simulink model "s_cd_hmc_v3_dsim"  (R2016b)
(part 2 of 59)

      mask help:
      | An explicitly laid-out delay line to avoid mapping to SRL16s
      | for use in pipelining to help achieve timing closure.
      mask init:
      | pipeline_init(gcb,'latency',latency);
      settings: AttributesFormatString=Latency = %<latency>
      mask Display:
      | port_label('input', 1, 'd');
      | port_label('output', 1, 'q');
      | disp(['Z^-', num2str(latency)]);
  pipeline6 : Subsystem  AncestorBlock=casper_library_delays/pipeline  mask(pipeline){latency=2}
      mask help:
      | An explicitly laid-out delay line to avoid mapping to SRL16s
      | for use in pipelining to help achieve timing closure.
      mask init:
      | pipeline_init(gcb,'latency',latency);
      settings: AttributesFormatString=Latency = %<latency>
      mask Display:
      | port_label('input', 1, 'd');
      | port_label('output', 1, 'q');
      | disp(['Z^-', num2str(latency)]);
  pipeline60 : Subsystem  AncestorBlock=casper_library_delays/pipeline  mask(pipeline){latency=2}
      mask help:
      | An explicitly laid-out delay line to avoid mapping to SRL16s
      | for use in pipelining to help achieve timing closure.
      mask init:
      | pipeline_init(gcb,'latency',latency);
      settings: AttributesFormatString=Latency = %<latency>
      mask Display:
      | port_label('input', 1, 'd');
      | port_label('output', 1, 'q');
      | disp(['Z^-', num2str(latency)]);
  pipeline61 : Subsystem  AncestorBlock=casper_library_delays/pipeline  mask(pipeline){latency=2}
      mask help:
      | An explicitly laid-out delay line to avoid mapping to SRL16s
      | for use in pipelining to help achieve timing closure.
      mask init:
      | pipeline_init(gcb,'latency',latency);
      settings: AttributesFormatString=Latency = %<latency>
      mask Display:
      | port_label('input', 1, 'd');
      | port_label('output', 1, 'q');
      | disp(['Z^-', num2str(latency)]);
  pipeline62 : Subsystem  AncestorBlock=casper_library_delays/pipeline  mask(pipeline){latency=3}
      mask help:
      | An explicitly laid-out delay line to avoid mapping to SRL16s
      | for use in pipelining to help achieve timing closure.
      mask init:
      | pipeline_init(gcb,'latency',latency);
      settings: AttributesFormatString=Latency = %<latency>
      mask Display:
      | port_label('input', 1, 'd');
      | port_label('output', 1, 'q');
      | disp(['Z^-', num2str(latency)]);
  pipeline63 : Subsystem  AncestorBlock=casper_library_delays/pipeline  mask(pipeline){latency=2}
      mask help:
      | An explicitly laid-out delay line to avoid mapping to SRL16s
      | for use in pipelining to help achieve timing closure.
      mask init:
      | pipeline_init(gcb,'latency',latency);
      settings: AttributesFormatString=Latency = %<latency>
      mask Display:
      | port_label('input', 1, 'd');
      | port_label('output', 1, 'q');
      | disp(['Z^-', num2str(latency)]);
  pipeline64 : Subsystem  AncestorBlock=casper_library_delays/pipeline  mask(pipeline){latency=2}
      mask help:
      | An explicitly laid-out delay line to avoid mapping to SRL16s
      | for use in pipelining to help achieve timing closure.
      mask init:
      | pipeline_init(gcb,'latency',latency);
      settings: AttributesFormatString=Latency = %<latency>
      mask Display:
      | port_label('input', 1, 'd');
      | port_label('output', 1, 'q');
      | disp(['Z^-', num2str(latency)]);
  pipeline65 : Subsystem  AncestorBlock=casper_library_delays/pipeline  mask(pipeline){latency=3}
      mask help:
      | An explicitly laid-out delay line to avoid mapping to SRL16s
      | for use in pipelining to help achieve timing closure.
      mask init:
      | pipeline_init(gcb,'latency',latency);
      settings: AttributesFormatString=Latency = %<latency>
      mask Display:
      | port_label('input', 1, 'd');
      | port_label('output', 1, 'q');
      | disp(['Z^-', num2str(latency)]);
  pipeline66 : Subsystem  AncestorBlock=casper_library_delays/pipeline  mask(pipeline){latency=2}
      mask help:
      | An explicitly laid-out delay line to avoid mapping to SRL16s
      | for use in pipelining to help achieve timing closure.
      mask init:
      | pipeline_init(gcb,'latency',latency);
      settings: AttributesFormatString=Latency = %<latency>
      mask Display:
      | port_label('input', 1, 'd');
      | port_label('output', 1, 'q');
      | disp(['Z^-', num2str(latency)]);
  pipeline67 : Subsystem  AncestorBlock=casper_library_delays/pipeline  mask(pipeline){latency=2}
      mask help:
      | An explicitly laid-out delay line to avoid mapping to SRL16s
      | for use in pipelining to help achieve timing closure.
      mask init:
      | pipeline_init(gcb,'latency',latency);
      settings: AttributesFormatString=Latency = %<latency>
      mask Display:
      | port_label('input', 1, 'd');
      | port_label('output', 1, 'q');
      | disp(['Z^-', num2str(latency)]);
  pipeline68 : Subsystem  AncestorBlock=casper_library_delays/pipeline  mask(pipeline){latency=2}
      mask help:
      | An explicitly laid-out delay line to avoid mapping to SRL16s
      | for use in pipelining to help achieve timing closure.
      mask init:
      | pipeline_init(gcb,'latency',latency);
      settings: AttributesFormatString=Latency = %<latency>
      mask Display:
      | port_label('input', 1, 'd');
      | port_label('output', 1, 'q');
      | disp(['Z^-', num2str(latency)]);
  pipeline69 : Subsystem  AncestorBlock=casper_library_delays/pipeline  mask(pipeline){latency=2}
      mask help:
      | An explicitly laid-out delay line to avoid mapping to SRL16s
      | for use in pipelining to help achieve timing closure.
      mask init:
      | pipeline_init(gcb,'latency',latency);
      settings: AttributesFormatString=Latency = %<latency>
      mask Display:
      | port_label('input', 1, 'd');
      | port_label('output', 1, 'q');
      | disp(['Z^-', num2str(latency)]);
  pipeline7 : Subsystem  AncestorBlock=casper_library_delays/pipeline  mask(pipeline){latency=2}
      mask help:
      | An explicitly laid-out delay line to avoid mapping to SRL16s
      | for use in pipelining to help achieve timing closure.
      mask init:
      | pipeline_init(gcb,'latency',latency);
      settings: AttributesFormatString=Latency = %<latency>
      mask Display:
      | port_label('input', 1, 'd');
      | port_label('output', 1, 'q');
      | disp(['Z^-', num2str(latency)]);
  pipeline70 : Subsystem  AncestorBlock=casper_library_delays/pipeline  mask(pipeline){latency=2}
      mask help:
      | An explicitly laid-out delay line to avoid mapping to SRL16s
      | for use in pipelining to help achieve timing closure.
      mask init:
      | pipeline_init(gcb,'latency',latency);
      settings: AttributesFormatString=Latency = %<latency>
      mask Display:
      | port_label('input', 1, 'd');
      | port_label('output', 1, 'q');
      | disp(['Z^-', num2str(latency)]);
  pipeline71 : Subsystem  AncestorBlock=casper_library_delays/pipeline  mask(pipeline){latency=2}
      mask help:
      | An explicitly laid-out delay line to avoid mapping to SRL16s
      | for use in pipelining to help achieve timing closure.
      mask init:
      | pipeline_init(gcb,'latency',latency);
      settings: AttributesFormatString=Latency = %<latency>
      mask Display:
      | port_label('input', 1, 'd');
      | port_label('output', 1, 'q');
      | disp(['Z^-', num2str(latency)]);
  pipeline72 : Subsystem  AncestorBlock=casper_library_delays/pipeline  mask(pipeline){latency=1}
      mask help:
      | An explicitly laid-out delay line to avoid mapping to SRL16s
      | for use in pipelining to help achieve timing closure.
      mask init:
      | pipeline_init(gcb,'latency',latency);
      settings: AttributesFormatString=Latency = %<latency>
      mask Display:
      | port_label('input', 1, 'd');
      | port_label('output', 1, 'q');
      | disp(['Z^-', num2str(latency)]);
  pipeline74 : Subsystem  AncestorBlock=casper_library_delays/pipeline  mask(pipeline){latency=2}
      mask help:
      | An explicitly laid-out delay line to avoid mapping to SRL16s
      | for use in pipelining to help achieve timing closure.
      mask init:
      | pipeline_init(gcb,'latency',latency);
      settings: AttributesFormatString=Latency = %<latency>
      mask Display:
      | port_label('input', 1, 'd');
      | port_label('output', 1, 'q');
      | disp(['Z^-', num2str(latency)]);
  pipeline75 : Subsystem  AncestorBlock=casper_library_delays/pipeline  mask(pipeline){latency=2}
      mask help:
      | An explicitly laid-out delay line to avoid mapping to SRL16s
      | for use in pipelining to help achieve timing closure.
      mask init:
      | pipeline_init(gcb,'latency',latency);
      settings: AttributesFormatString=Latency = %<latency>
      mask Display:
      | port_label('input', 1, 'd');
      | port_label('output', 1, 'q');
      | disp(['Z^-', num2str(latency)]);
  pipeline76 : Subsystem  AncestorBlock=casper_library_delays/pipeline  mask(pipeline){latency=2}
      mask help:
      | An explicitly laid-out delay line to avoid mapping to SRL16s
      | for use in pipelining to help achieve timing closure.
      mask init:
      | pipeline_init(gcb,'latency',latency);
      settings: AttributesFormatString=Latency = %<latency>
      mask Display:
      | port_label('input', 1, 'd');
      | port_label('output', 1, 'q');
      | disp(['Z^-', num2str(latency)]);
  pipeline79 : Subsystem  AncestorBlock=casper_library_delays/pipeline  mask(pipeline){latency=2}
      mask help:
      | An explicitly laid-out delay line to avoid mapping to SRL16s
      | for use in pipelining to help achieve timing closure.
      mask init:
      | pipeline_init(gcb,'latency',latency);
      settings: AttributesFormatString=Latency = %<latency>
      mask Display:
      | port_label('input', 1, 'd');
      | port_label('output', 1, 'q');
      | disp(['Z^-', num2str(latency)]);
  pipeline8 : Subsystem  AncestorBlock=casper_library_delays/pipeline  mask(pipeline){latency=2}
      mask help:
      | An explicitly laid-out delay line to avoid mapping to SRL16s
      | for use in pipelining to help achieve timing closure.
      mask init:
      | pipeline_init(gcb,'latency',latency);
      settings: AttributesFormatString=Latency = %<latency>
      mask Display:
      | port_label('input', 1, 'd');
      | port_label('output', 1, 'q');
      | disp(['Z^-', num2str(latency)]);
  pipeline80 : Subsystem  AncestorBlock=casper_library_delays/pipeline  mask(pipeline){latency=2}
      mask help:
      | An explicitly laid-out delay line to avoid mapping to SRL16s
      | for use in pipelining to help achieve timing closure.
      mask init:
      | pipeline_init(gcb,'latency',latency);
      settings: AttributesFormatString=Latency = %<latency>
      mask Display:
      | port_label('input', 1, 'd');
      | port_label('output', 1, 'q');
      | disp(['Z^-', num2str(latency)]);
  pipeline81 : Subsystem  AncestorBlock=casper_library_delays/pipeline  mask(pipeline){latency=2}
      mask help:
      | An explicitly laid-out delay line to avoid mapping to SRL16s
      | for use in pipelining to help achieve timing closure.
      mask init:
      | pipeline_init(gcb,'latency',latency);
      settings: AttributesFormatString=Latency = %<latency>
      mask Display:
      | port_label('input', 1, 'd');
      | port_label('output', 1, 'q');
      | disp(['Z^-', num2str(latency)]);
  pipeline82 : Subsystem  AncestorBlock=casper_library_delays/pipeline  mask(pipeline){latency=2}
      mask help:
      | An explicitly laid-out delay line to avoid mapping to SRL16s
      | for use in pipelining to help achieve timing closure.
      mask init:
      | pipeline_init(gcb,'latency',latency);
      settings: AttributesFormatString=Latency = %<latency>
      mask Display:
      | port_label('input', 1, 'd');
      | port_label('output', 1, 'q');
      | disp(['Z^-', num2str(latency)]);
  pipeline83 : Subsystem  AncestorBlock=casper_library_delays/pipeline  mask(pipeline){latency=2}
      mask help:
      | An explicitly laid-out delay line to avoid mapping to SRL16s
      | for use in pipelining to help achieve timing closure.
      mask init:
      | pipeline_init(gcb,'latency',latency);
      settings: AttributesFormatString=Latency = %<latency>
      mask Display:
      | port_label('input', 1, 'd');
      | port_label('output', 1, 'q');
      | disp(['Z^-', num2str(latency)]);
  pipeline85 : Subsystem  AncestorBlock=casper_library_delays/pipeline  mask(pipeline){latency=2}
      mask help:
      | An explicitly laid-out delay line to avoid mapping to SRL16s
      | for use in pipelining to help achieve timing closure.
      mask init:
      | pipeline_init(gcb,'latency',latency);
      settings: AttributesFormatString=Latency = %<latency>
      mask Display:
      | port_label('input', 1, 'd');
      | port_label('output', 1, 'q');
      | disp(['Z^-', num2str(latency)]);
  pipeline86 : Subsystem  AncestorBlock=casper_library_delays/pipeline  mask(pipeline){latency=2}
      mask help:
      | An explicitly laid-out delay line to avoid mapping to SRL16s
      | for use in pipelining to help achieve timing closure.
      mask init:
      | pipeline_init(gcb,'latency',latency);
      settings: AttributesFormatString=Latency = %<latency>
      mask Display:
      | port_label('input', 1, 'd');
      | port_label('output', 1, 'q');
      | disp(['Z^-', num2str(latency)]);
  pipeline87 : Subsystem  AncestorBlock=casper_library_delays/pipeline  mask(pipeline){latency=2}
      mask help:
      | An explicitly laid-out delay line to avoid mapping to SRL16s
      | for use in pipelining to help achieve timing closure.
      mask init:
      | pipeline_init(gcb,'latency',latency);
      settings: AttributesFormatString=Latency = %<latency>
      mask Display:
      | port_label('input', 1, 'd');
      | port_label('output', 1, 'q');
      | disp(['Z^-', num2str(latency)]);
  pipeline9 : Subsystem  AncestorBlock=casper_library_delays/pipeline  mask(pipeline){latency=2}
      mask help:
      | An explicitly laid-out delay line to avoid mapping to SRL16s
      | for use in pipelining to help achieve timing closure.
      mask init:
      | pipeline_init(gcb,'latency',latency);
      settings: AttributesFormatString=Latency = %<latency>
      mask Display:
      | port_label('input', 1, 'd');
      | port_label('output', 1, 'q');
      | disp(['Z^-', num2str(latency)]);
  pipeline90 : Subsystem  AncestorBlock=casper_library_delays/pipeline  mask(pipeline){latency=2}
      mask help:
      | An explicitly laid-out delay line to avoid mapping to SRL16s
      | for use in pipelining to help achieve timing closure.
      mask init:
      | pipeline_init(gcb,'latency',latency);
      settings: AttributesFormatString=Latency = %<latency>
      mask Display:
      | port_label('input', 1, 'd');
      | port_label('output', 1, 'q');
      | disp(['Z^-', num2str(latency)]);
  pipeline91 : Subsystem  AncestorBlock=casper_library_delays/pipeline  mask(pipeline){latency=2}
      mask help:
      | An explicitly laid-out delay line to avoid mapping to SRL16s
      | for use in pipelining to help achieve timing closure.
      mask init:
      | pipeline_init(gcb,'latency',latency);
      settings: AttributesFormatString=Latency = %<latency>
      mask Display:
      | port_label('input', 1, 'd');
      | port_label('output', 1, 'q');
      | disp(['Z^-', num2str(latency)]);
  pipeline92 : Subsystem  AncestorBlock=casper_library_delays/pipeline  mask(pipeline){latency=2}
      mask help:
      | An explicitly laid-out delay line to avoid mapping to SRL16s
      | for use in pipelining to help achieve timing closure.
      mask init:
      | pipeline_init(gcb,'latency',latency);
      settings: AttributesFormatString=Latency = %<latency>
      mask Display:
      | port_label('input', 1, 'd');
      | port_label('output', 1, 'q');
      | disp(['Z^-', num2str(latency)]);
  pipeline93 : Subsystem  AncestorBlock=casper_library_delays/pipeline  mask(pipeline){latency=2}
      mask help:
      | An explicitly laid-out delay line to avoid mapping to SRL16s
      | for use in pipelining to help achieve timing closure.
      mask init:
      | pipeline_init(gcb,'latency',latency);
      settings: AttributesFormatString=Latency = %<latency>
      mask Display:
      | port_label('input', 1, 'd');
      | port_label('output', 1, 'q');
      | disp(['Z^-', num2str(latency)]);
  pipeline94 : Subsystem  AncestorBlock=casper_library_delays/pipeline  mask(pipeline){latency=2}
      mask help:
      | An explicitly laid-out delay line to avoid mapping to SRL16s
      | for use in pipelining to help achieve timing closure.
      mask init:
      | pipeline_init(gcb,'latency',latency);
      settings: AttributesFormatString=Latency = %<latency>
      mask Display:
      | port_label('input', 1, 'd');
      | port_label('output', 1, 'q');
      | disp(['Z^-', num2str(latency)]);
  pipeline95 : Subsystem  AncestorBlock=casper_library_delays/pipeline  mask(pipeline){latency=2}
      mask help:
      | An explicitly laid-out delay line to avoid mapping to SRL16s
      | for use in pipelining to help achieve timing closure.
      mask init:
      | pipeline_init(gcb,'latency',latency);
      settings: AttributesFormatString=Latency = %<latency>
      mask Display:
      | port_label('input', 1, 'd');
      | port_label('output', 1, 'q');
      | disp(['Z^-', num2str(latency)]);
  pipeline96 : Subsystem  AncestorBlock=casper_library_delays/pipeline  mask(pipeline){latency=2}
      mask help:
      | An explicitly laid-out delay line to avoid mapping to SRL16s
      | for use in pipelining to help achieve timing closure.
      mask init:
      | pipeline_init(gcb,'latency',latency);
      settings: AttributesFormatString=Latency = %<latency>
      mask Display:
      | port_label('input', 1, 'd');
      | port_label('output', 1, 'q');
      | disp(['Z^-', num2str(latency)]);
  pipeline97 : Subsystem  AncestorBlock=casper_library_delays/pipeline  mask(pipeline){latency=2}
      mask help:
      | An explicitly laid-out delay line to avoid mapping to SRL16s
      | for use in pipelining to help achieve timing closure.
      mask init:
      | pipeline_init(gcb,'latency',latency);
      settings: AttributesFormatString=Latency = %<latency>
      mask Display:
      | port_label('input', 1, 'd');
      | port_label('output', 1, 'q');
      | disp(['Z^-', num2str(latency)]);
  pipeline98 : Subsystem  AncestorBlock=casper_library_delays/pipeline  mask(pipeline){latency=2}
      mask help:
      | An explicitly laid-out delay line to avoid mapping to SRL16s
      | for use in pipelining to help achieve timing closure.
      mask init:
      | pipeline_init(gcb,'latency',latency);
      settings: AttributesFormatString=Latency = %<latency>
      mask Display:
      | port_label('input', 1, 'd');
      | port_label('output', 1, 'q');
      | disp(['Z^-', num2str(latency)]);
  pipeline99 : Subsystem  AncestorBlock=casper_library_delays/pipeline  mask(pipeline){latency=2}
      mask help:
      | An explicitly laid-out delay line to avoid mapping to SRL16s
      | for use in pipelining to help achieve timing closure.
      mask init:
      | pipeline_init(gcb,'latency',latency);
      settings: AttributesFormatString=Latency = %<latency>
      mask Display:
      | port_label('input', 1, 'd');
      | port_label('output', 1, 'q');
      | disp(['Z^-', num2str(latency)]);
  reorder_status : Subsystem  Tag=xps:sw_reg  AncestorBlock=xps_library/software_register  mask(swreg){io_dir=To Processor, io_delay=0, sample_period=1, names=[timestep_err_cnt receive_err_cnt discard_cnt relock_err_cnt overflow_err_cnt], bitwidths=5, bin_pts=0, arith_types=0, sim_port=off, show_format=on}
      mask prompts: io_dir "I/O direction"; io_delay "I/O delay"; sample_period "Sample period"; names "Bitfield names [msb...lsb]"; bitwidths "Bitfield widths"; bin_pts "Bitfield binary pts"; arith_types "Bitfield types, ufix=0, fix=1, bool=2"; sim_port "Provide sim input/output?"; show_format "Print format string?"
      mask help: A 32-bit software-accessible register. Can be divided into bitfields of varying widths and types using the fields in the block mask.
      mask init:
      | swreg_init(gcb)
      settings: AttributesFormatString=5 outputs:uf5.0,uf5.0,uf5.0,uf5.0,uf5.0 = 25 bits
      mask TypeOptions io_dir: To Processor | From Processor
      mask Callback io_dir:
      | mask_enables = get_param(gcb, 'MaskEnables');
      | mask_names = get_param(gcb, 'MaskNames');
      | if strcmp(get_param(gcb, 'io_dir'), 'To Processor'),
      |     mask_enables{ismember(mask_names, 'sample_period')} = 'off';
      | else
      |     mask_enables{ismember(mask_names, 'sample_period')} = 'on';
      | end
      | set_param(gcb, 'MaskEnables', mask_enables);
  rx_dest_ip : Subsystem  Tag=xps:sw_reg  AncestorBlock=xps_library/software register  mask(swreg){io_dir=To Processor, io_delay=0, sample_period=1, names=reg, bitwidths=32, bin_pts=0, arith_types=0, sim_port=off, show_format=on}
      mask prompts: io_dir "I/O direction"; io_delay "I/O delay"; sample_period "Sample period"; names "Bitfield names [msb...lsb]"; bitwidths "Bitfield widths"; bin_pts "Bitfield binary pts"; arith_types "Bitfield types, ufix=0, fix=1, bool=2"; sim_port "Provide sim input/output?"; show_format "Print format string?"
      mask help: A 32-bit software-accessible register. Can be divided into bitfields of varying widths and types using the fields in the block mask.
      mask init:
      | swreg_init(gcb)
      settings: AttributesFormatString=1output:uf32.0 = 32 bits
      mask TypeOptions io_dir: To Processor | From Processor
      mask Callback io_dir:
      | mask_enables = get_param(gcb, 'MaskEnables');
      | mask_names = get_param(gcb, 'MaskNames');
      | if strcmp(get_param(gcb, 'io_dir'), 'To Processor'),
      |     mask_enables{ismember(mask_names, 'sample_period')} = 'off';
      | else
      |     mask_enables{ismember(mask_names, 'sample_period')} = 'on';
      | end
      | set_param(gcb, 'MaskEnables', mask_enables);
  rx_dest_port : Subsystem  Tag=xps:sw_reg  AncestorBlock=xps_library/software register  mask(swreg){io_dir=To Processor, io_delay=0, sample_period=1, names=reg, bitwidths=16, bin_pts=0, arith_types=0, sim_port=off, show_format=on}
      mask prompts: io_dir "I/O direction"; io_delay "I/O delay"; sample_period "Sample period"; names "Bitfield names [msb...lsb]"; bitwidths "Bitfield widths"; bin_pts "Bitfield binary pts"; arith_types "Bitfield types, ufix=0, fix=1, bool=2"; sim_port "Provide sim input/output?"; show_format "Print format string?"
      mask help: A 32-bit software-accessible register. Can be divided into bitfields of varying widths and types using the fields in the block mask.
      mask init:
      | swreg_init(gcb)
      settings: AttributesFormatString=1output:uf16.0 = 16 bits
      mask TypeOptions io_dir: To Processor | From Processor
      mask Callback io_dir:
      | mask_enables = get_param(gcb, 'MaskEnables');
      | mask_names = get_param(gcb, 'MaskNames');
      | if strcmp(get_param(gcb, 'io_dir'), 'To Processor'),
      |     mask_enables{ismember(mask_names, 'sample_period')} = 'off';
      | else
      |     mask_enables{ismember(mask_names, 'sample_period')} = 'on';
      | end
      | set_param(gcb, 'MaskEnables', mask_enables);
  rx_src_ip : Subsystem  Tag=xps:sw_reg  AncestorBlock=xps_library/software register  mask(swreg){io_dir=To Processor, io_delay=0, sample_period=1, names=reg, bitwidths=32, bin_pts=0, arith_types=0, sim_port=off, show_format=on}
      mask prompts: io_dir "I/O direction"; io_delay "I/O delay"; sample_period "Sample period"; names "Bitfield names [msb...lsb]"; bitwidths "Bitfield widths"; bin_pts "Bitfield binary pts"; arith_types "Bitfield types, ufix=0, fix=1, bool=2"; sim_port "Provide sim input/output?"; show_format "Print format string?"
      mask help: A 32-bit software-accessible register. Can be divided into bitfields of varying widths and types using the fields in the block mask.
      mask init:
      | swreg_init(gcb)
      settings: AttributesFormatString=1output:uf32.0 = 32 bits
      mask TypeOptions io_dir: To Processor | From Processor
      mask Callback io_dir:
      | mask_enables = get_param(gcb, 'MaskEnables');
      | mask_names = get_param(gcb, 'MaskNames');
      | if strcmp(get_param(gcb, 'io_dir'), 'To Processor'),
      |     mask_enables{ismember(mask_names, 'sample_period')} = 'off';
      | else
      |     mask_enables{ismember(mask_names, 'sample_period')} = 'on';
      | end
      | set_param(gcb, 'MaskEnables', mask_enables);
  rx_src_port : Subsystem  Tag=xps:sw_reg  AncestorBlock=xps_library/software register  mask(swreg){io_dir=To Processor, io_delay=0, sample_period=1, names=reg, bitwidths=16, bin_pts=0, arith_types=0, sim_port=off, show_format=on}
      mask prompts: io_dir "I/O direction"; io_delay "I/O delay"; sample_period "Sample period"; names "Bitfield names [msb...lsb]"; bitwidths "Bitfield widths"; bin_pts "Bitfield binary pts"; arith_types "Bitfield types, ufix=0, fix=1, bool=2"; sim_port "Provide sim input/output?"; show_format "Print format string?"
      mask help: A 32-bit software-accessible register. Can be divided into bitfields of varying widths and types using the fields in the block mask.
      mask init:
      | swreg_init(gcb)
      settings: AttributesFormatString=1output:uf16.0 = 16 bits
      mask TypeOptions io_dir: To Processor | From Processor
      mask Callback io_dir:
      | mask_enables = get_param(gcb, 'MaskEnables');
      | mask_names = get_param(gcb, 'MaskNames');
      | if strcmp(get_param(gcb, 'io_dir'), 'To Processor'),
      |     mask_enables{ismember(mask_names, 'sample_period')} = 'off';
      | else
      |     mask_enables{ismember(mask_names, 'sample_period')} = 'on';
      | end
      | set_param(gcb, 'MaskEnables', mask_enables);
  snap_adc0 : Subsystem  Tag=casper:bitsnap  AncestorBlock=casper_library_scopes/bitfield snapshot  mask(bitsnap){io_names=[d0 d1 d2 d3 d4 d5 d6 d7 dv sync], io_widths=[10 10 10 10 10 10 10 10 1 1], io_bps=[9 9 9 9 9 9 9 9 0 0], io_types=[1 1 1 1 1 1 1 1 2 2], snap_storage=bram, snap_dram_dimm=2, snap_dram_clock=250, snap_nsamples=11, snap_data_width=128, snap_offset=on, snap_circap=off, snap_value=off, snap_use_dsp48=off, snap_delay=0, extra_names=[c d], extra_widths=[30 2], extra_bps=[0 0], extra_types=[0 0]}
      mask prompts: io_names "Names [msb...lsb]"; io_widths "Widths [msb...lsb]"; io_bps "Binary pts [msb...lsb]"; io_types "Data types [msb...lsb], ufix=0, fix=1, bool=2"; snap_storage "Storage medium"; snap_dram_dimm "DRAM dimm"; snap_dram_clock "DRAM clock rate"; snap_nsamples "Number of Samples (2^?)"; snap_data_width "Data width"; snap_offset "Start delay support"; snap_circap "Circular capture support"; snap_value "Extra value capture support"; snap_use_dsp48 "Use DSP48s to implement counters"; snap_delay "Pre-snapshot delay"; extra_names "Names [msb...lsb]"; extra_widths "Widths [msb...lsb]"; extra_bps "Binary pts [msb...lsb]"; extra_types "Data types [msb...lsb], ufix=0, fix=1, bool=2"
      mask help:
      | A wrapped snapshot block. Allows specification of inputs to a snapblock word so the toolflow can automatically set up the scope.
      | See documentation for snapshot for explanation of parameters.
      mask init:
      | bitsnap_init(gcb);
      mask TypeOptions snap_storage: bram | dram
      mask Callback snap_storage: bitsnap_callback();
      mask TypeOptions snap_dram_dimm: 1 | 2 | 3 | 4
      mask TypeOptions snap_dram_clock: 200 | 250 | 266 | 300 | 333
      mask TypeOptions snap_data_width: 8 | 16 | 32 | 64 | 128
      mask Callback snap_value: bitsnap_callback();
  snap_adc1 : Subsystem  Tag=casper:bitsnap  AncestorBlock=casper_library_scopes/bitfield snapshot  mask(bitsnap){io_names=[d0 d1 d2 d3 d4 d5 d6 d7 dv sync], io_widths=[10 10 10 10 10 10 10 10 1 1], io_bps=[9 9 9 9 9 9 9 9 0 0], io_types=[1 1 1 1 1 1 1 1 2 2], snap_storage=bram, snap_dram_dimm=2, snap_dram_clock=250, snap_nsamples=11, snap_data_width=128, snap_offset=on, snap_circap=off, snap_value=off, snap_use_dsp48=off, snap_delay=0, extra_names=[c d], extra_widths=[30 2], extra_bps=[0 0], extra_types=[0 0]}
      mask prompts: io_names "Names [msb...lsb]"; io_widths "Widths [msb...lsb]"; io_bps "Binary pts [msb...lsb]"; io_types "Data types [msb...lsb], ufix=0, fix=1, bool=2"; snap_storage "Storage medium"; snap_dram_dimm "DRAM dimm"; snap_dram_clock "DRAM clock rate"; snap_nsamples "Number of Samples (2^?)"; snap_data_width "Data width"; snap_offset "Start delay support"; snap_circap "Circular capture support"; snap_value "Extra value capture support"; snap_use_dsp48 "Use DSP48s to implement counters"; snap_delay "Pre-snapshot delay"; extra_names "Names [msb...lsb]"; extra_widths "Widths [msb...lsb]"; extra_bps "Binary pts [msb...lsb]"; extra_types "Data types [msb...lsb], ufix=0, fix=1, bool=2"
      mask help:
      | A wrapped snapshot block. Allows specification of inputs to a snapblock word so the toolflow can automatically set up the scope.
      | See documentation for snapshot for explanation of parameters.
      mask init:
      | bitsnap_init(gcb);
      mask TypeOptions snap_storage: bram | dram
      mask Callback snap_storage: bitsnap_callback();
      mask TypeOptions snap_dram_dimm: 1 | 2 | 3 | 4
      mask TypeOptions snap_dram_clock: 200 | 250 | 266 | 300 | 333
      mask TypeOptions snap_data_width: 8 | 16 | 32 | 64 | 128
      mask Callback snap_value: bitsnap_callback();
  spead_status : Subsystem  Tag=xps:sw_reg  AncestorBlock=xps_library/software_register  mask(swreg){io_dir=To Processor, io_delay=0, sample_period=1, names=[magic_err_cnt header_err_cnt pad_err_cnt pkt_len_err_cnt pkt_cnt], bitwidths=6, bin_pts=0, arith_types=0, sim_port=off, show_format=on}
      mask prompts: io_dir "I/O direction"; io_delay "I/O delay"; sample_period "Sample period"; names "Bitfield names [msb...lsb]"; bitwidths "Bitfield widths"; bin_pts "Bitfield binary pts"; arith_types "Bitfield types, ufix=0, fix=1, bool=2"; sim_port "Provide sim input/output?"; show_format "Print format string?"
      mask help: A 32-bit software-accessible register. Can be divided into bitfields of varying widths and types using the fields in the block mask.
      mask init:
      | swreg_init(gcb)
      settings: AttributesFormatString=5 outputs:uf6.0,uf6.0,uf6.0,uf6.0,uf6.0 = 30 bits
      mask TypeOptions io_dir: To Processor | From Processor
      mask Callback io_dir:
      | mask_enables = get_param(gcb, 'MaskEnables');
      | mask_names = get_param(gcb, 'MaskNames');
      | if strcmp(get_param(gcb, 'io_dir'), 'To Processor'),
      |     mask_enables{ismember(mask_names, 'sample_period')} = 'off';
      | else
      |     mask_enables{ismember(mask_names, 'sample_period')} = 'on';
      | end
      | set_param(gcb, 'MaskEnables', mask_enables);
  sync_gen : Subsystem  mask{zerolsbs=((15 + 1) + 8)}
      mask prompts: zerolsbs "No. LSBs to be zero:"
  sys_rst_cnt : Subsystem  Tag=xps:sw_reg  AncestorBlock=xps_library/software register  mask(swreg){io_dir=To Processor, io_delay=0, sample_period=1, names=cnt, bitwidths=32, bin_pts=0, arith_types=0, sim_port=off, show_format=on}
      mask prompts: io_dir "I/O direction"; io_delay "I/O delay"; sample_period "Sample period"; names "Bitfield names [msb...lsb]"; bitwidths "Bitfield widths"; bin_pts "Bitfield binary pts"; arith_types "Bitfield types, ufix=0, fix=1, bool=2"; sim_port "Provide sim input/output?"; show_format "Print format string?"
      mask help: A 32-bit software-accessible register. Can be divided into bitfields of varying widths and types using the fields in the block mask.
      mask init:
      | swreg_init(gcb)
      settings: AttributesFormatString=1output:uf32.0 = 32 bits
      mask TypeOptions io_dir: To Processor | From Processor
      mask Callback io_dir:
      | mask_enables = get_param(gcb, 'MaskEnables');
      | mask_names = get_param(gcb, 'MaskNames');
      | if strcmp(get_param(gcb, 'io_dir'), 'To Processor'),
      |     mask_enables{ismember(mask_names, 'sample_period')} = 'off';
      | else
      |     mask_enables{ismember(mask_names, 'sample_period')} = 'on';
      | end
      | set_param(gcb, 'MaskEnables', mask_enables);
  time_gen1 : Subsystem  mask{n_bits_period=fft_stages-1-2-1+8, n_bits_increment=0, n_bits_counter=48-(fft_stages+8)}
      mask prompts: n_bits_period "Period (2^?)"; n_bits_increment "Increment (2^?)"; n_bits_counter "Counter size (2^?)"
  time_gen_cd : Subsystem  mask{n_bits_period=fft_stages-1-2, n_bits_increment=0, n_bits_counter=48-fft_stages}
      mask prompts: n_bits_period "Period (2^?)"; n_bits_increment "Increment (2^?)"; n_bits_counter "Counter size (2^?)"
  time_rst_cnt : Subsystem  Tag=xps:sw_reg  AncestorBlock=xps_library/software register  mask(swreg){io_dir=To Processor, io_delay=0, sample_period=1, names=cnt, bitwidths=32, bin_pts=0, arith_types=0, sim_port=off, show_format=on}
      mask prompts: io_dir "I/O direction"; io_delay "I/O delay"; sample_period "Sample period"; names "Bitfield names [msb...lsb]"; bitwidths "Bitfield widths"; bin_pts "Bitfield binary pts"; arith_types "Bitfield types, ufix=0, fix=1, bool=2"; sim_port "Provide sim input/output?"; show_format "Print format string?"
      mask help: A 32-bit software-accessible register. Can be divided into bitfields of varying widths and types using the fields in the block mask.
      mask init:
      | swreg_init(gcb)
      settings: AttributesFormatString=1output:uf32.0 = 32 bits
      mask TypeOptions io_dir: To Processor | From Processor
      mask Callback io_dir:
      | mask_enables = get_param(gcb, 'MaskEnables');
      | mask_names = get_param(gcb, 'MaskNames');
      | if strcmp(get_param(gcb, 'io_dir'), 'To Processor'),
      |     mask_enables{ismember(mask_names, 'sample_period')} = 'off';
      | else
      |     mask_enables{ismember(mask_names, 'sample_period')} = 'on';
      | end
      | set_param(gcb, 'MaskEnables', mask_enables);
  tl_cd0 : Subsystem  mask(timed_latch){n_bits_time=48-fft_stages, n_bits_quantization=fft_stages, n_bits_counters=4}
      mask prompts: n_bits_time "Number bits in time to compare"; n_bits_quantization "Time offset from lsb"; n_bits_counters "Bits in status counters"
      mask help:
      | Latches load_value when armed and current_time matches requested time.
      | current_time should be in ADC samples.
      mask init:
      | set_param([gcb,'/status'], 'bitwidths', mat2str([1, repmat(n_bits_counters, 1, 2)]));
      mask Help:
      | When armed, will latch new value when current time matches the time
      | specified. The input time should be in samples and mask settings allow
      | a portion of this to be compared to cater for quantization. Arm and latch
      | counts allow the current state, pending and missed latch events to be
      | determined.
  tl_cd0_control : Subsystem  Tag=xps:sw_reg  AncestorBlock=xps_library/software_register  mask(swreg){io_dir=From Processor, io_delay=0, sample_period=1, names=[arm load_immediate load_time_msw], bitwidths=[1 1 16], bin_pts=[0 0 0], arith_types=[2 2 0], sim_port=on, show_format=on}
      mask prompts: io_dir "I/O direction"; io_delay "I/O delay"; sample_period "Sample period"; names "Bitfield names [msb...lsb]"; bitwidths "Bitfield widths"; bin_pts "Bitfield binary pts"; arith_types "Bitfield types, ufix=0, fix=1, bool=2"; sim_port "Provide sim input/output?"; show_format "Print format string?"
      mask help: A 32-bit software-accessible register. Can be divided into bitfields of varying widths and types using the fields in the block mask.
      mask init:
      | swreg_init(gcb)
      settings: AttributesFormatString=3 inputs:b,b,uf16.0 = 18 bits
      mask TypeOptions io_dir: To Processor | From Processor
      mask Callback io_dir:
      | mask_enables = get_param(gcb, 'MaskEnables');
      | mask_names = get_param(gcb, 'MaskNames');
      | if strcmp(get_param(gcb, 'io_dir'), 'To Processor'),
      |     mask_enables{ismember(mask_names, 'sample_period')} = 'off';
      | else
      |     mask_enables{ismember(mask_names, 'sample_period')} = 'on';
      | end
      | set_param(gcb, 'MaskEnables', mask_enables);
  tl_cd0_control_lsw : Subsystem  Tag=xps:sw_reg  AncestorBlock=xps_library/software_register  mask(swreg){io_dir=From Processor, io_delay=0, sample_period=1, names=load_time_lsw, bitwidths=32, bin_pts=0, arith_types=0, sim_port=on, show_format=on}
      mask prompts: io_dir "I/O direction"; io_delay "I/O delay"; sample_period "Sample period"; names "Bitfield names [msb...lsb]"; bitwidths "Bitfield widths"; bin_pts "Bitfield binary pts"; arith_types "Bitfield types, ufix=0, fix=1, bool=2"; sim_port "Provide sim input/output?"; show_format "Print format string?"
      mask help: A 32-bit software-accessible register. Can be divided into bitfields of varying widths and types using the fields in the block mask.
      mask init:
      | swreg_init(gcb)
      settings: AttributesFormatString=1input:uf32.0 = 32 bits
      mask TypeOptions io_dir: To Processor | From Processor
      mask Callback io_dir:
      | mask_enables = get_param(gcb, 'MaskEnables');
      | mask_names = get_param(gcb, 'MaskNames');
      | if strcmp(get_param(gcb, 'io_dir'), 'To Processor'),
      |     mask_enables{ismember(mask_names, 'sample_period')} = 'off';
      | else
      |     mask_enables{ismember(mask_names, 'sample_period')} = 'on';
      | end
      | set_param(gcb, 'MaskEnables', mask_enables);
  tl_cd1 : Subsystem  mask(timed_latch){n_bits_time=48-fft_stages, n_bits_quantization=fft_stages, n_bits_counters=4}
      mask prompts: n_bits_time "Number bits in time to compare"; n_bits_quantization "Time offset from lsb"; n_bits_counters "Bits in status counters"
      mask help:
      | Latches load_value when armed and current_time matches requested time.
      | current_time should be in ADC samples.
      mask init:
      | set_param([gcb,'/status'], 'bitwidths', mat2str([1, repmat(n_bits_counters, 1, 2)]));
      mask Help:
      | When armed, will latch new value when current time matches the time
      | specified. The input time should be in samples and mask settings allow
      | a portion of this to be compared to cater for quantization. Arm and latch
      | counts allow the current state, pending and missed latch events to be
      | determined.
  tl_cd1_control : Subsystem  Tag=xps:sw_reg  AncestorBlock=xps_library/software_register  mask(swreg){io_dir=From Processor, io_delay=0, sample_period=1, names=[arm load_immediate load_time_msw], bitwidths=[1 1 16], bin_pts=[0 0 0], arith_types=[2 2 0], sim_port=on, show_format=on}
      mask prompts: io_dir "I/O direction"; io_delay "I/O delay"; sample_period "Sample period"; names "Bitfield names [msb...lsb]"; bitwidths "Bitfield widths"; bin_pts "Bitfield binary pts"; arith_types "Bitfield types, ufix=0, fix=1, bool=2"; sim_port "Provide sim input/output?"; show_format "Print format string?"
      mask help: A 32-bit software-accessible register. Can be divided into bitfields of varying widths and types using the fields in the block mask.
      mask init:
      | swreg_init(gcb)
      settings: AttributesFormatString=3 inputs:b,b,uf16.0 = 18 bits
      mask TypeOptions io_dir: To Processor | From Processor
      mask Callback io_dir:
      | mask_enables = get_param(gcb, 'MaskEnables');
      | mask_names = get_param(gcb, 'MaskNames');
      | if strcmp(get_param(gcb, 'io_dir'), 'To Processor'),
      |     mask_enables{ismember(mask_names, 'sample_period')} = 'off';
      | else
      |     mask_enables{ismember(mask_names, 'sample_period')} = 'on';
      | end
      | set_param(gcb, 'MaskEnables', mask_enables);
  tl_cd1_control_lsw : Subsystem  Tag=xps:sw_reg  AncestorBlock=xps_library/software_register  mask(swreg){io_dir=From Processor, io_delay=0, sample_period=1, names=load_time_lsw, bitwidths=32, bin_pts=0, arith_types=0, sim_port=on, show_format=on}
      mask prompts: io_dir "I/O direction"; io_delay "I/O delay"; sample_period "Sample period"; names "Bitfield names [msb...lsb]"; bitwidths "Bitfield widths"; bin_pts "Bitfield binary pts"; arith_types "Bitfield types, ufix=0, fix=1, bool=2"; sim_port "Provide sim input/output?"; show_format "Print format string?"
      mask help: A 32-bit software-accessible register. Can be divided into bitfields of varying widths and types using the fields in the block mask.
      mask init:
      | swreg_init(gcb)
      settings: AttributesFormatString=1input:uf32.0 = 32 bits
      mask TypeOptions io_dir: To Processor | From Processor
      mask Callback io_dir:
      | mask_enables = get_param(gcb, 'MaskEnables');
      | mask_names = get_param(gcb, 'MaskNames');
      | if strcmp(get_param(gcb, 'io_dir'), 'To Processor'),
      |     mask_enables{ismember(mask_names, 'sample_period')} = 'off';
      | else
      |     mask_enables{ismember(mask_names, 'sample_period')} = 'on';
      | end
      | set_param(gcb, 'MaskEnables', mask_enables);
  tl_cd_bs0 : Subsystem  mask(timed_latch){n_bits_time=48-fft_stages, n_bits_quantization=fft_stages, n_bits_counters=4}
      mask prompts: n_bits_time "Number bits in time to compare"; n_bits_quantization "Time offset from lsb"; n_bits_counters "Bits in status counters"
      mask help:
      | Latches load_value when armed and current_time matches requested time.
      | current_time should be in ADC samples.
      mask init:
      | set_param([gcb,'/status'], 'bitwidths', mat2str([1, repmat(n_bits_counters, 1, 2)]));
      mask Help:
      | When armed, will latch new value when current time matches the time
      | specified. The input time should be in samples and mask settings allow
      | a portion of this to be compared to cater for quantization. Arm and latch
      | counts allow the current state, pending and missed latch events to be
      | determined.
  tl_cd_bs1 : Subsystem  mask(timed_latch){n_bits_time=48-fft_stages, n_bits_quantization=fft_stages, n_bits_counters=4}
      mask prompts: n_bits_time "Number bits in time to compare"; n_bits_quantization "Time offset from lsb"; n_bits_counters "Bits in status counters"
      mask help:
      | Latches load_value when armed and current_time matches requested time.
      | current_time should be in ADC samples.
      mask init:
      | set_param([gcb,'/status'], 'bitwidths', mat2str([1, repmat(n_bits_counters, 1, 2)]));
      mask Help:
      | When armed, will latch new value when current time matches the time
      | specified. The input time should be in samples and mask settings allow
      | a portion of this to be compared to cater for quantization. Arm and latch
      | counts allow the current state, pending and missed latch events to be
      | determined.
  trig_time_lsw : Subsystem  Tag=xps:sw_reg  AncestorBlock=xps_library/software register  mask(swreg){io_dir=From Processor, io_delay=0, sample_period=1, names=lsw, bitwidths=32, bin_pts=0, arith_types=0, sim_port=off, show_format=on}
      mask prompts: io_dir "I/O direction"; io_delay "I/O delay"; sample_period "Sample period"; names "Bitfield names [msb...lsb]"; bitwidths "Bitfield widths"; bin_pts "Bitfield binary pts"; arith_types "Bitfield types, ufix=0, fix=1, bool=2"; sim_port "Provide sim input/output?"; show_format "Print format string?"
      mask help: A 32-bit software-accessible register. Can be divided into bitfields of varying widths and types using the fields in the block mask.
      mask init:
      | swreg_init(gcb)
      settings: AttributesFormatString=1input:uf32.0 = 32 bits
      mask TypeOptions io_dir: To Processor | From Processor
      mask Callback io_dir:
      | mask_enables = get_param(gcb, 'MaskEnables');
      | mask_names = get_param(gcb, 'MaskNames');
      | if strcmp(get_param(gcb, 'io_dir'), 'To Processor'),
      |     mask_enables{ismember(mask_names, 'sample_period')} = 'off';
      | else
      |     mask_enables{ismember(mask_names, 'sample_period')} = 'on';
      | end
      | set_param(gcb, 'MaskEnables', mask_enables);
  trig_time_msw : Subsystem  Tag=xps:sw_reg  AncestorBlock=xps_library/software register  mask(swreg){io_dir=From Processor, io_delay=0, sample_period=1, names=msw, bitwidths=16, bin_pts=0, arith_types=0, sim_port=off, show_format=on}
      mask prompts: io_dir "I/O direction"; io_delay "I/O delay"; sample_period "Sample period"; names "Bitfield names [msb...lsb]"; bitwidths "Bitfield widths"; bin_pts "Bitfield binary pts"; arith_types "Bitfield types, ufix=0, fix=1, bool=2"; sim_port "Provide sim input/output?"; show_format "Print format string?"
      mask help: A 32-bit software-accessible register. Can be divided into bitfields of varying widths and types using the fields in the block mask.
      mask init:
      | swreg_init(gcb)
      settings: AttributesFormatString=1input:uf16.0 = 16 bits
      mask TypeOptions io_dir: To Processor | From Processor
      mask Callback io_dir:
      | mask_enables = get_param(gcb, 'MaskEnables');
      | mask_names = get_param(gcb, 'MaskNames');
      | if strcmp(get_param(gcb, 'io_dir'), 'To Processor'),
      |     mask_enables{ismember(mask_names, 'sample_period')} = 'off';
      | else
      |     mask_enables{ismember(mask_names, 'sample_period')} = 'on';
      | end
      | set_param(gcb, 'MaskEnables', mask_enables);
  tvg : Subsystem
  tx_metadata : Subsystem  Tag=xps:sw_reg  AncestorBlock=xps_library/software register  mask(swreg){io_dir=From Processor, io_delay=0, sample_period=1, names=[porttx board_id], bitwidths=16, bin_pts=0, arith_types=0, sim_port=off, show_format=on}
      mask prompts: io_dir "I/O direction"; io_delay "I/O delay"; sample_period "Sample period"; names "Bitfield names [msb...lsb]"; bitwidths "Bitfield widths"; bin_pts "Bitfield binary pts"; arith_types "Bitfield types, ufix=0, fix=1, bool=2"; sim_port "Provide sim input/output?"; show_format "Print format string?"
      mask help: A 32-bit software-accessible register. Can be divided into bitfields of varying widths and types using the fields in the block mask.
      mask init:
      | swreg_init(gcb)
      settings: AttributesFormatString=2 inputs:uf16.0,uf16.0 = 32 bits
      mask TypeOptions io_dir: To Processor | From Processor
      mask Callback io_dir:
      | mask_enables = get_param(gcb, 'MaskEnables');
      | mask_names = get_param(gcb, 'MaskNames');
      | if strcmp(get_param(gcb, 'io_dir'), 'To Processor'),
      |     mask_enables{ismember(mask_names, 'sample_period')} = 'off';
      | else
      |     mask_enables{ismember(mask_names, 'sample_period')} = 'on';
      | end
      | set_param(gcb, 'MaskEnables', mask_enables);
  unpack_and_reorder : Subsystem
  up_timestep_er_cnt : Subsystem  Tag=xps:sw_reg  AncestorBlock=xps_library/software register  mask(swreg){io_dir=To Processor, io_delay=0, sample_period=1, names=cnt, bitwidths=32, bin_pts=0, arith_types=0, sim_port=off, show_format=on}
      mask prompts: io_dir "I/O direction"; io_delay "I/O delay"; sample_period "Sample period"; names "Bitfield names [msb...lsb]"; bitwidths "Bitfield widths"; bin_pts "Bitfield binary pts"; arith_types "Bitfield types, ufix=0, fix=1, bool=2"; sim_port "Provide sim input/output?"; show_format "Print format string?"
      mask help: A 32-bit software-accessible register. Can be divided into bitfields of varying widths and types using the fields in the block mask.
      mask init:
      | swreg_init(gcb)
      settings: AttributesFormatString=1output:uf32.0 = 32 bits
      mask TypeOptions io_dir: To Processor | From Processor
      mask Callback io_dir:
      | mask_enables = get_param(gcb, 'MaskEnables');
      | mask_names = get_param(gcb, 'MaskNames');
      | if strcmp(get_param(gcb, 'io_dir'), 'To Processor'),
      |     mask_enables{ismember(mask_names, 'sample_period')} = 'off';
      | else
      |     mask_enables{ismember(mask_names, 'sample_period')} = 'on';
      | end
      | set_param(gcb, 'MaskEnables', mask_enables);
  wb_prog_delay : Subsystem  mask{n_bits_fft=fft_stages, n_bits_cd=17}
      mask prompts: n_bits_fft "fft length (2^?)"; n_bits_cd "max coarse delay (2^?)"
  wb_prog_delay1 : Subsystem  mask{n_bits_fft=fft_stages, n_bits_cd=17}
      mask prompts: n_bits_fft "fft length (2^?)"; n_bits_cd "max coarse delay (2^?)"
  x_setup : Subsystem  Tag=xps:sw_reg  AncestorBlock=xps_library/software_register  mask(swreg){io_dir=From Processor, io_delay=0, sample_period=1, names=[f_per_x ip_per_x num_x snap_arm stop_mux pktstart_mux], bitwidths=[13 6 9 1 2 1], bin_pts=[0 4 0 0 0 0], arith_types=[0 0 0 2 0 0], sim_port=off, show_format=on}
      mask prompts: io_dir "I/O direction"; io_delay "I/O delay"; sample_period "Sample period"; names "Bitfield names [msb...lsb]"; bitwidths "Bitfield widths"; bin_pts "Bitfield binary pts"; arith_types "Bitfield types, ufix=0, fix=1, bool=2"; sim_port "Provide sim input/output?"; show_format "Print format string?"
      mask help: A 32-bit software-accessible register. Can be divided into bitfields of varying widths and types using the fields in the block mask.
      mask init:
      | swreg_init(gcb)
      settings: AttributesFormatString=6 inputs:uf13.0,uf6.4,uf9.0,b,uf2.0,uf1.0 = 32 bits
      mask TypeOptions io_dir: To Processor | From Processor
      mask Callback io_dir:
      | mask_enables = get_param(gcb, 'MaskEnables');
      | mask_names = get_param(gcb, 'MaskNames');
      | if strcmp(get_param(gcb, 'io_dir'), 'To Processor'),
      |     mask_enables{ismember(mask_names, 'sample_period')} = 'off';
      | else
      |     mask_enables{ismember(mask_names, 'sample_period')} = 'on';
      | end
      | set_param(gcb, 'MaskEnables', mask_enables);
      mask DialogControl ParameterTabVar0 Prompt: Setup
  xsg_core_config : Subsystem  Tag=xps:xsg  AncestorBlock=xps_library/XSG_core_config  mask(xsg core config){hw_sys=SKARAB:xc7vx690t, clk_src=sys_clk, clk_rate=238, sample_period=1, synthesis_tool=XST}
      mask prompts: hw_sys "Hardware Platform"; clk_src "User IP Clock source"; clk_rate "User IP Clock Rate (MHz)"; sample_period "Sample Period"; synthesis_tool "Synthesis Tool:"
      mask help:
      | The XSG Core Config block is used to configure the System Generator design
      | for the casper_xps toolflow. Settings here are used to configure the
      | Xilinx System Generator block parameters automatically, and control toolflow
      | script  execution. It needs to be at the top level of all designs being compiled
      | with the casper_xps toolflow.
      mask init:
      | xps_xsg_conf_mask;
      mask Help: eval('xlWeb([getenv(''MLIB_ROOT''), ''\doc\html\sys_xsg_core_config\sys_xsg_core_config.html''])')
      mask TypeOptions hw_sys: ROACH:sx95t | ROACH:lx110t | ROACH2:sx475t | SNAP:xc7k160t | KC705:xc7k325t | SKARAB:xc7vx690t
      mask Callback hw_sys: xps_xsg_conf_callback
      mask TypeOptions clk_src: sys_clk | aux_clk
      mask Callback clk_src: xps_xsg_conf_callback
      mask Callback clk_rate: xps_xsg_conf_callback
      mask TypeOptions synthesis_tool: Leonardo Spectrum | Synplify | Synplify Pro | XST
      mask Display: fprintf(['MSSGE\n', hw_sys]);
  tag scope: cnt_rst=global, flag_pktstart=global, pktstart_sel=global, sys_rst=global, up_timestep_error=global
  wires:
  Constant3/1 -> gbe0/8(rx_overrun_ack)
  Constant4/1 -> gbe0/7(rx_ack)
  [gbe_rst] -> pipeline99/1(d)
  unpack_and_reorder/5(recvd) -> pipeline17/1(d)
  sync_gen/2(dout) -> bus_expand6/1(bus_in)
  sync_gen/3(dvalid) -> Gateway Out5/1, impulse_gen0/6(en), impulse_gen1/6(en)
  Slice4/1 -> pipeline16/1(d)
  pipeline16/1(q) -> local_time_lsw/1(out_timestamp_lsw)
  Slice16/1 -> Convert6/1
  pipeline47/1(q) -> local_time_msw/1(out_timestamp_msw)
  Convert6/1 -> pipeline47/1(d)
  [time80_48] -> Slice16/1, Slice4/1
  Concat22/1 -> [ld_val0]
  Concat3/1 -> [ld_val1]
  bus_expand17/1(msb_out2) -> [unpack_recvd0]
  bus_expand17/2(lsb_out1) -> [unpack_recvd1]
  Slice12/1 -> Gateway Out6/1, [time80]
  impulse_gen0/1(sync_out) -> Gateway Out2/1, [sync80]
  impulse_gen0/2(dout) -> [d80_adc0]
  impulse_gen0/4(misco) -> [time80_48], Slice12/1
  impulse_gen1/1(sync_out) -> Terminator6/1
  impulse_gen1/2(dout) -> [d80_adc1]
  impulse_gen1/3(dvalid) -> Terminator8/1
  impulse_gen1/4(misco) -> [dig_flags]
  impulse0/1(in_offset) -> Slice7/1
  impulse0/2(in_amplitude) -> impulse_gen0/3(impulse_amplitude)
  impulse1/1(in_offset) -> Slice8/1
  impulse1/2(in_amplitude) -> impulse_gen1/3(impulse_amplitude)
  sync_gen/1(sync) -> Gateway Out4/1, impulse_gen0/4(sync_in), impulse_gen1/4(sync_in)
  bus_expand6/1(msb_out2) -> impulse_gen0/5(din)
  bus_expand6/2(lsb_out1) -> impulse_gen1/5(din)
  sync_gen/5(misco) -> impulse_gen1/7(misci)
  sync_gen/4(time_out) -> impulse_gen0/7(misci)
  Constant31/1 -> Concat9/2
  [unpack_timestamp] -> Concat9/1
  [up_timestep_error] -> Logical15/1
  [sys_rst] -> Logical15/2
  Logical15/1 -> edge_detect17/1(in)
  edge_detect17/1(out) -> [sys_relock]
  phase0/1(in_initial) -> Reinterpret2/1
  delta_delay0/1(in_delta) -> Reinterpret1/1
  phase0/2(in_delta) -> Reinterpret3/1
  [sys_relock] -> sync_gen/5(relock)
  [unpack_d160] -> sync_gen/3(din)
  Slice7/1 -> impulse_gen0/2(impulse_offset)
  Slice8/1 -> impulse_gen1/2(impulse_offset)
  Reinterpret8/1 -> Concat22/1
  Reinterpret1/1 -> Concat22/2
  Reinterpret2/1 -> Concat22/3
  Reinterpret3/1 -> Concat22/4
  phase1/1(in_initial) -> Reinterpret5/1
  delta_delay1/1(in_delta) -> Reinterpret4/1
  phase1/2(in_delta) -> Reinterpret6/1
  Reinterpret4/1 -> Concat3/2
  Reinterpret5/1 -> Concat3/3
  Reinterpret6/1 -> Concat3/4
  Reinterpret7/1 -> Concat3/1
  delay0/1(in_initial) -> Reinterpret8/1
  delay1/1(in_initial) -> Reinterpret7/1
  trig_time_msw/1(in_msw) -> pipeline28/1(d)
  trig_time_lsw/1(in_lsw) -> pipeline44/1(d)
  Concat13/1 -> Relational10/1
  pipeline28/1(q) -> Concat13/1
  pipeline44/1(q) -> Concat13/2
  [valid80] -> Counter/2
  [sync80] -> Counter/1
  Constant12/1 -> Relational7/2
  Counter/1 -> Relational7/1
  Relational10/1 -> Mux/2
  Relational7/1 -> Mux/3
  [valid80] -> Delay49/1
  Logical12/1 -> Logical14/1
  Logical14/1 -> [adc_snap_trig]
  [adc_snap_arm] -> Logical14/2
  [time80_48] -> Relational10/2
  Delay49/1 -> Logical12/2
  Mux/1 -> Logical12/1
  [adc_snap_trig_source] -> Mux/1
  iptx_base/1(in_reg) -> pipeline105/1(d)
  pipeline105/1(q) -> [tx_ip_base]
  tx_metadata/1(in_porttx) -> pipeline106/1(d)
  tx_metadata/2(in_board_id) -> pipeline107/1(d)
  pipeline106/1(q) -> [tx_port]
  pipeline107/1(q) -> [tx_board_id]
  edge_detect4/1(out) -> pipeline5/1(d)
  control/6(in_cnt_rst) -> edge_detect1/1(in)
  edge_detect1/1(out) -> pipeline14/1(d)
  control/3(in_gbe_rst) -> pipeline6/1(d)
  control/1(in_sys_rst) -> pipeline3/1(d)
  pipeline3/1(q) -> [sys_rst]
  pipeline5/1(q) -> [clr_status]
  pipeline6/1(q) -> [gbe_rst]
  pipeline7/1(q) -> [gbe_txen]
  pipeline13/1(q) -> [tvg_adc_en]
  pipeline14/1(q) -> [cnt_rst]
  control/5(in_tvg_adc) -> pipeline13/1(d)
  edge_detect2/1(out) -> pipeline38/1(d)
  pipeline38/1(q) -> [gbe_cnt_rst]
  control/7(in_gbe_cnt_rst) -> edge_detect2/1(in)
  control/4(in_gbe_txen) -> pipeline7/1(d)
  control/2(in_status_clr) -> edge_detect4/1(in)
  pipeline43/1(q) -> [adc_snap_arm]
  control/8(in_adc_snap_arm) -> pipeline43/1(d)
  control/9(in_adc_snap_trig_select) -> pipeline39/1(d)
  pipeline39/1(q) -> [adc_snap_trig_source]
  [gbe_cnt_rst] -> pipeline31/1(d)
  pipeline31/1(q) -> gbe0/9(debug_rst)
  gbe0/13(rx_dest_ip) -> pipeline115/1(d)
  gbe0/14(rx_dest_port) -> pipeline116/1(d)
  [rx_dest_ip] -> pipeline/1(d)
  pipeline/1(q) -> rx_dest_ip/1(out_reg)
  [rx_dest_port] -> pipeline18/1(d)
  pipeline18/1(q) -> rx_dest_port/1(out_reg)
  gbe0/1(led_up) -> pipeline100/1(d)
  [forty_gbe_led_up] -> pipeline19/1(d)
  gbe0/2(led_rx) -> pipeline101/1(d)
  [forty_gbe_led_rx] -> pipeline20/1(d)
  gbe0/3(led_tx) -> pipeline102/1(d)
  [forty_gbe_led_tx] -> pipeline51/1(d)
  gbe0/4(tx_afull) -> pipeline103/1(d)
  gbe0/5(tx_overflow) -> pipeline104/1(d)
  gbe0/12(rx_overrun) -> pipeline114/1(d)
  pipeline19/1(q) -> gbe_status/1(out_led_up)
  pipeline20/1(q) -> gbe_status/2(out_led_rx)
  pipeline51/1(q) -> gbe_status/3(out_led_tx)
  gbe0/8(rx_source_ip) -> pipeline110/1(d)
  gbe0/9(rx_source_port) -> pipeline111/1(d)
  pipeline55/1(q) -> rx_src_ip/1(out_reg)
  pipeline56/1(q) -> rx_src_port/1(out_reg)
  [forty_gbe_rx_src_port] -> pipeline56/1(d)
  [forty_gbe_rx_src_ip] -> pipeline55/1(d)
  gbe0/6(rx_data) -> pipeline108/1(d)
  gbe0/7(rx_valid) -> pipeline109/1(d)
  gbe0/10(rx_end_of_frame) -> pipeline112/1(d)
  gbe0/11(rx_bad_frame) -> pipeline113/1(d)
  pipeline80/1(q) -> [flag_sync]
  pipeline81/1(q) -> [flag_misc]
  pipeline82/1(q) -> [flag_dvalid]
  pipeline83/1(q) -> [flag_time]
  pipeline85/1(q) -> time_gen1/4(rd_sync_in)
  pipeline87/1(q) -> time_gen1/6(rd_misc_in)
  Constant44/1 -> concat2/2
  [flag_time] -> concat2/1
  pack/5(destination_ip) -> [s256_ip]
  pack/6(destination_port) -> [s256_port]
  [flag_sync] -> pack/1(sync_in)
  [flag_dvalid] -> pack/2(en)
  [flag_misc] -> pack/3(din)
  concat2/1 -> pack/4(timestamp)
  [tx_board_id] -> pack/5(board_id)
  [tx_ip_base] -> pack/6(base_ip)
  [tx_port] -> pack/7(base_port)
  Constant32/1 -> pack/10(ips_per_destination)
  Constant30/1 -> pack/9(n_destinations)
  Constant28/1 -> pack/8(step_size)
  pack/7(sync) -> Terminator58/1
  pack/1(dout) -> [s256_d]
  [s256_d] -> pipeline98/1(d)
  [s256_ip] -> pipeline97/1(d)
  [s256_port] -> pipeline96/1(d)
  Logical2/1 -> gbe0/6(tx_end_of_frame)
  [s256_v] -> Logical1/2
  [s256_eof] -> Logical2/2
  Delay1/1 -> Logical1/1, Logical2/1
  [s256_eof] -> Delay1/2
  pipeline96/1(q) -> gbe0/5(tx_dest_port)
  pipeline97/1(q) -> gbe0/4(tx_dest_ip)
  pipeline98/1(q) -> gbe0/2(tx_data)
  pipeline99/1(q) -> gbe0/1(rst)
  [gbe_txen] -> Delay1/1
  pack/2(dvalid) -> [s256_v]
  pack/3(eof) -> [s256_eof]
  pack/4(overflow) -> [s256_of]
  pipeline100/1(q) -> [forty_gbe_led_up]
  pipeline101/1(q) -> [forty_gbe_led_rx]
  pipeline102/1(q) -> [forty_gbe_led_tx]
  pipeline103/1(q) -> [forty_gbe_tx_full]
  pipeline104/1(q) -> [forty_gbe_tx_of]
  pipeline108/1(q) -> [forty_gbe_rx_data]
  pipeline110/1(q) -> [forty_gbe_rx_src_ip]
  pipeline111/1(q) -> [forty_gbe_rx_src_port]
  pipeline112/1(q) -> [forty_gbe_rx_eof]
  pipeline113/1(q) -> [forty_gbe_rx_bad]
  pipeline114/1(q) -> [forty_gbe_rx_overrun]
  pipeline115/1(q) -> [rx_dest_ip]
  pipeline116/1(q) -> [rx_dest_port]
  [forty_gbe_rx_data] -> unpack_and_reorder/1(d256)
  [forty_gbe_rx_valid] -> unpack_and_reorder/2(dv256)
  [forty_gbe_rx_eof] -> unpack_and_reorder/3(eof256)
  pipeline109/1(q) -> [forty_gbe_rx_valid]
  unpack_and_reorder/6(flags) -> Terminator9/1
  unpack_and_reorder/2(d160) -> pipeline11/1(d)
  unpack_and_reorder/3(dv) -> pipeline12/1(d)
  unpack_and_reorder/4(time) -> pipeline15/1(d)
  unpack_and_reorder/1(sync) -> pipeline10/1(d)
  Inverter1/1 -> Logical6/1
  [unpack_recvd0] -> Inverter1/1
  [unpack_dv] -> Logical6/2
  Inverter2/1 -> Logical7/1
  [unpack_recvd1] -> Inverter2/1
  [unpack_dv] -> Logical7/2
  Logical7/1 -> Logical/2
  Logical6/1 -> Logical/1
  Logical/1 -> [unpack_missing]
  pipeline10/1(q) -> [unpack_sync]
  pipeline11/1(q) -> [unpack_d160]
  pipeline12/1(q) -> [unpack_dv]
  pipeline15/1(q) -> [unpack_timestamp]
  pipeline17/1(q) -> bus_expand17/1(bus_in)
  [up_dbg_rst] -> Subsystem4/1(rst)
  [upg_sp_dv] -> Logical3/2
  [upg_sp_eof] -> Logical3/1
  [upg_reo_time] -> Subsystem1/3(time)
  [upg_reo_recv] -> Subsystem1/4(recv)
  [upg_reo_dv] -> Subsystem1/2(dv)
  [up_dbg_rst] -> Subsystem1/1(rst)
  Subsystem1/6(time_change) -> [reo_time_change]
  Logical5/1 -> Subsystem1/7(overflow_err)
  [upg_of80_p1] -> Logical5/2
  [upg_of80_p0] -> Logical5/1
  [upg_sperr_magic] -> Subsystem4/2(in0)
  [upg_sperr_len] -> Subsystem4/5(in3)
  [upg_sperr_hdr] -> Subsystem4/3(in1)
  [upg_sperr_pad] -> Subsystem4/4(in2)
  Delay/1 -> pipeline85/1(d)  "gapsync"
  Delay3/1 -> pipeline86/1(d)  "gapdata"
  Mux1/1 -> pipeline87/1(d)  "gapvalid"
  Subsystem4/5(out4) -> spead_status/5(out_pkt_cnt)
  Logical3/1 -> Subsystem4/6(in4)
  Constant1/1 -> sync_gen/4(misci)
  [q_sync] -> time_gen1/1(wr_sync_in)
  [q_dv] -> time_gen1/2(wr_en)
  [time80] -> Slice2/1
  pipeline86/1(q) -> time_gen1/5(rd_en)
  time_gen1/1(rd_sync_out) -> pipeline80/1(d)
  time_gen1/4(rd_misc_out) -> pipeline81/1(d)
  time_gen1/2(rd_dvalid) -> pipeline82/1(d)
  time_gen1/3(rd_val_out) -> pipeline83/1(d)
  Slice2/1 -> time_gen1/3(wr_val_in)
  [d80_adc1] -> pipeline62/1(d)
  [d80_adc0] -> pipeline57/1(d)
  bus_expand1/1(msb_out8) -> Gateway Out8/1, snap_adc0/1(in_d0)
  bus_expand1/2(out7) -> Gateway Out10/1, snap_adc0/2(in_d1)
  bus_expand1/3(out6) -> Gateway Out11/1, snap_adc0/3(in_d2)
  bus_expand1/4(out5) -> Gateway Out12/1, snap_adc0/4(in_d3)
  bus_expand1/5(out4) -> Gateway Out13/1, snap_adc0/5(in_d4)
  bus_expand1/6(out3) -> Gateway Out14/1, snap_adc0/6(in_d5)
  bus_expand1/7(out2) -> Gateway Out15/1, snap_adc0/7(in_d6)
  bus_expand1/8(lsb_out1) -> Gateway Out16/1, snap_adc0/8(in_d7)
  pipeline57/1(q) -> bus_expand1/1(bus_in)
  pipeline62/1(q) -> bus_expand2/1(bus_in)
  [valid80] -> pipeline27/1(d), pipeline65/1(d)
  [adc_snap_trig] -> pipeline29/1(d), Gateway Out1/1, snap_adc0/12(trig), snap_adc1/12(trig)
  Logical1/1 -> gbe0/3(tx_valid)
  pipeline59/1(q) -> [ct_tvg_en]
  control/10(in_ct_tvg_en) -> pipeline59/1(d)
  pipeline65/1(q) -> Gateway Out/1, snap_adc0/11(we), snap_adc1/11(we)
  pipeline52/1(q) -> [up_dbg_rst]
  control/11(in_unpack_debug_reset) -> pipeline52/1(d)
  Subsystem1/7(timestep_err) -> [up_timestep_error]
  Subsystem4/4(out3) -> spead_status/4(out_pkt_len_err_cnt)
  Subsystem4/3(out2) -> spead_status/3(out_pad_err_cnt)
  Subsystem4/2(out1) -> spead_status/2(out_header_err_cnt)
  Subsystem4/1(out0) -> spead_status/1(out_magic_err_cnt)
  [upg_reo_disc] -> Subsystem1/5(discard_err)
  [upg_reo_relock] -> Subsystem1/6(relock_err)
  Subsystem1/1(timestep_err_cnt) -> reorder_status/1(out_timestep_err_cnt)
  Subsystem1/2(recv_err_cnt) -> reorder_status/2(out_receive_err_cnt)
  Subsystem1/3(discard_err_cnt) -> reorder_status/3(out_discard_cnt)
  Subsystem1/4(relock_err_cnt) -> reorder_status/4(out_relock_err_cnt)
  Subsystem1/5(overflow_err_cnt) -> reorder_status/5(out_overflow_err_cnt)
  Subsystem2/1(out0) -> cd_status/1(out_hmc_err_cnt)
  Subsystem2/2(out1) -> cd_status/2(out_pol0_parity_err_cnt)
  Subsystem2/3(out2) -> cd_status/3(out_pol1_parity_err_cnt)
  [hmc_parity_pol0] -> Subsystem2/4(in2), Subsystem2/3(in1)
  [clr_status] -> Subsystem2/1(rst)
  [hmc_error] -> Subsystem2/2(in0)
  [ct_tvg_en2] -> Mux1/1
  [ct_dv] -> Delay5/1
  Delay6/1 -> Mux1/2
  Delay7/1 -> tvg/1(In1), Delay/1
  [ct_sync] -> Delay7/1
  [ct_d256] -> Delay6/1
  Delay5/1 -> tvg/2(In2), Delay3/1
  tl_cd0_control/3(in_load_time_msw) -> Concat6/1
  tl_cd0_control_lsw/1(in_load_time_lsw) -> Concat6/2
  Constant42/1 -> tl_cd0_control_lsw/1(sim_1)
  Constant40/1 -> tl_cd0_control/3(sim_3)
  Constant41/1 -> tl_cd0_control/2(sim_2)
  Constant43/1 -> Delay12/1
  Delay12/1 -> tl_cd0_control/1(sim_1)
  Concat6/1 -> [tl_cd0_load_time]
  tl_cd0_control/2(in_load_immediate) -> [tl_cd0_load_immediate]
  tl_cd0_control/1(in_arm) -> [tl_cd0_arm]
  tl_cd1_control/3(in_load_time_msw) -> Concat8/1
  tl_cd1_control_lsw/1(in_load_time_lsw) -> Concat8/2
  Constant47/1 -> tl_cd1_control_lsw/1(sim_1)
  Constant45/1 -> tl_cd1_control/3(sim_3)
  Constant46/1 -> tl_cd1_control/2(sim_2)
  Constant48/1 -> Delay13/1
  Delay13/1 -> tl_cd1_control/1(sim_1)
  Concat8/1 -> [tl_cd1_load_time]
  tl_cd1_control/2(in_load_immediate) -> [tl_cd1_load_immediate]
  tl_cd1_control/1(in_arm) -> [tl_cd1_arm]
  [ld_val0] -> pipeline23/1(d)
  [clr_status] -> pipeline142/1(d), pipeline25/1(d)
  tl_cd0/6(time) -> [time80_tl_cd0]
  Constant6/1 -> Concat15/2
  Concat15/1 -> pipeline141/1(d), Gateway Out7/1, pipeline24/1(d)
  [time80] -> Concat15/1
  pipeline25/1(q) -> tl_cd0/1(rst)
  pipeline24/1(q) -> tl_cd0/2(current_time)
  pipeline23/1(q) -> tl_cd0/3(load_value)
  pipeline22/1(q) -> tl_cd0/4(sync_in)
  pipeline21/1(q) -> tl_cd0/5(din)
  pipeline26/1(q) -> tl_cd0/6(en)
  [sync80] -> pipeline147/1(d), pipeline22/1(d)
  [valid80] -> pipeline145/1(d), pipeline26/1(d)
  Constant16/1 -> tl_cd0/7(misci)
  tl_cd0/7(misco) -> Terminator/1
  tl_cd0/3(sync_out) -> [sync_tl_cd0]
  tl_cd0/5(dvalid) -> [dvalid_tl_cd0]
  tl_cd0/4(dout) -> [dout_tl_cd0]
  tl_cd0/2(enable) -> [en_tl_cd0]
  tl_cd0/1(value) -> [delay_tl_cd0]
  pipeline76/1(q) -> tl_cd0/10(load_time)
  pipeline75/1(q) -> tl_cd0/9(load_immediate)
  pipeline74/1(q) -> tl_cd0/8(arm)
  [tl_cd0_arm] -> pipeline74/1(d)
  [tl_cd0_load_immediate] -> pipeline75/1(d)
  [tl_cd0_load_time] -> pipeline76/1(d)
  tvg/1(Out1) -> Mux1/3
  pipeline121/1(q) -> [f_per_x]
  pipeline124/1(q) -> [ip_per_x]
  pipeline125/1(q) -> [num_x]
  x_setup/1(in_f_per_x) -> pipeline121/1(d)
  x_setup/2(in_ip_per_x) -> pipeline124/1(d)
  x_setup/3(in_num_x) -> pipeline125/1(d)
  pipeline120/1(q) -> [pack_snap_arm]
  x_setup/4(in_snap_arm) -> pipeline120/1(d)
  pipeline2/1(q) -> gbe_in_msb/1(in_d_msb)
  pipeline122/1(q) -> gbe_in_lsb/1(in_d_lsb)
  [s256_ip] -> pipeline123/1(d)
  [s256_port] -> pipeline117/1(d)
  [s256_eof] -> pipeline118/1(d)
  [s256_v] -> pipeline119/1(d)
  pipeline118/1(q) -> gbe_in_misc/4(in_eof)
  pipeline119/1(q) -> gbe_in_misc/3(in_valid_raw)
  [s256_d] -> Slice3/1, Slice1/1
  Slice1/1 -> pipeline2/1(d)
  Slice3/1 -> pipeline122/1(d)
  [pack_snap_arm] -> Logical9/1, Logical8/1
  [s256_v] -> Logical8/2
  [s256_eof] -> Logical9/2
  Logical8/1 -> gbe_in_msb/2(we), gbe_in_lsb/2(we), gbe_in_misc/8(we)
  Logical9/1 -> gbe_in_misc/9(trig), gbe_in_lsb/3(trig), gbe_in_msb/3(trig)
  pipeline117/1(q) -> gbe_in_misc/2(in_src_port)
  pipeline123/1(q) -> gbe_in_misc/1(in_src_ip)
  Mux2/1 -> pipeline8/1(d)
  pipeline8/1(q) -> gbe_in_lsb/4(stop), gbe_in_misc/10(stop), gbe_in_msb/4(stop)
  [forty_gbe_tx_of] -> pipeline9/1(d)
  [forty_gbe_tx_full] -> pipeline58/1(d)
  pipeline9/1(q) -> gbe_in_misc/6(in_gbe_of)
  pipeline58/1(q) -> gbe_in_misc/5(in_gbe_full)
  [debug_stop_mux] -> Mux2/1
  x_setup/5(in_stop_mux) -> pipeline63/1(d)
  pipeline63/1(q) -> [debug_stop_mux]
  [forty_gbe_tx_err] -> pipeline64/1(d)
  pipeline64/1(q) -> gbe_in_misc/7(in_gbe_err)
  Logical11/1 -> Mux2/2
  [forty_gbe_tx_of] -> Logical11/3, Mux2/3
  [forty_gbe_tx_full] -> Logical11/2, Mux2/4
  [forty_gbe_tx_err] -> Logical11/1, Mux2/5
  [packin_rdy] -> pipeline66/1(d)
  [packin_dv] -> pipeline79/1(d)
  [packin_heapid] -> pipeline94/1(d)
  [packin_heapsize] -> pipeline95/1(d)
  [packin_heapoffset] -> pipeline126/1(d)
  [packin_boardid] -> pipeline127/1(d)
  [packin_freqbase] -> pipeline128/1(d)
  pipeline66/1(q) -> pack_inputs/1(in_data_ready)
  pipeline79/1(q) -> pack_inputs/9(trig), pack_inputs/8(we), pack_inputs/2(in_data_valid)
  pipeline94/1(q) -> pack_inputs/3(in_heap_id)
  pipeline95/1(q) -> pack_inputs/4(in_heap_size)
  pipeline126/1(q) -> pack_inputs/5(in_heap_offset)
  pipeline127/1(q) -> pack_inputs/6(in_board_id)
  pipeline128/1(q) -> pack_inputs/7(in_frequency_base)
  pipeline129/1(q) -> [flag_pktstart]
  [ct_pktstart] -> pipeline129/1(d)
  pipeline130/1(q) -> [pktstart_sel]
  x_setup/6(in_pktstart_mux) -> pipeline130/1(d)
  Constant/1 -> [ct_sync]
  Constant2/1 -> [ct_dv]
  Constant5/1 -> [ct_d256]
  Constant7/1 -> [ct_tvg_en2]
  Constant10/1 -> [ct_pktstart]
  Constant11/1 -> [q_sync]
  Constant13/1 -> [q_dv]
  Gateway Out/1 -> To Workspace/1
  Gateway Out1/1 -> To Workspace1/1
  Gateway Out2/1 -> To Workspace2/1
  Gateway Out3/1 -> To Workspace3/1
  impulse_gen0/3(dvalid) -> [valid80], Gateway Out3/1
  Constant14/1 -> impulse0/1(sim_1)
  Constant15/1 -> impulse0/2(sim_2)
  Constant18/1 -> impulse1/1(sim_1)
  Constant19/1 -> impulse1/2(sim_2)
  Gateway Out4/1 -> To Workspace4/1
  Gateway Out5/1 -> To Workspace5/1
  Gateway Out6/1 -> To Workspace6/1
  Gateway Out7/1 -> To Workspace7/1
  Gateway Out8/1 -> To Workspace8/1
  Gateway Out10/1 -> To Workspace10/1
  Gateway Out11/1 -> To Workspace11/1
  Gateway Out12/1 -> To Workspace12/1
  Gateway Out13/1 -> To Workspace13/1
  Gateway Out14/1 -> To Workspace14/1
  Gateway Out15/1 -> To Workspace15/1
  Gateway Out16/1 -> To Workspace16/1
  Constant22/1 -> delay0/1(sim_1)
  Constant23/1 -> delay1/1(sim_1)
  Gateway Out70/1 -> To Workspace72/1
  Gateway Out71/1 -> To Workspace71/1
  Gateway Out64/1 -> To Workspace70/1
  Gateway Out65/1 -> To Workspace68/1
  Gateway Out66/1 -> To Workspace67/1
  Gateway Out67/1 -> To Workspace66/1
  Gateway Out69/1 -> To Workspace69/1
  Gateway Out68/1 -> To Workspace65/1
  bus_expand13/8(lsb_out1) -> Gateway Out70/1
  bus_expand13/7(out2) -> Gateway Out71/1
  bus_expand13/6(out3) -> Gateway Out64/1
  bus_expand13/5(out4) -> Gateway Out65/1
  bus_expand13/4(out5) -> Gateway Out66/1
  bus_expand13/3(out6) -> Gateway Out67/1
  bus_expand13/2(out7) -> Gateway Out68/1
  bus_expand13/1(msb_out8) -> Gateway Out69/1
  [d80_adc0] -> pipeline21/1(d)
  bus_expand2/1(msb_out8) -> snap_adc1/1(in_d0)
  bus_expand2/2(out7) -> snap_adc1/2(in_d1)
  bus_expand2/3(out6) -> snap_adc1/3(in_d2)
  bus_expand2/4(out5) -> snap_adc1/4(in_d3)
  bus_expand2/5(out4) -> snap_adc1/5(in_d4)
  bus_expand2/6(out3) -> snap_adc1/6(in_d5)
  bus_expand2/7(out2) -> snap_adc1/7(in_d6)
  bus_expand2/8(lsb_out1) -> snap_adc1/8(in_d7)
  pipeline29/1(q) -> snap_adc0/10(in_sync), snap_adc1/10(in_sync)
  pipeline27/1(q) -> snap_adc0/9(in_dv), snap_adc1/9(in_dv)
  Concat9/1 -> sync_gen/1(time_in)
  [unpack_dv] -> sync_gen/2(en)
  [up_timestep_error] -> Counter3/1
  [sys_rst] -> Counter4/1
  Counter3/1 -> pipeline30/1(d)
  Counter4/1 -> pipeline32/1(d)
  pipeline30/1(q) -> up_timestep_er_cnt/1(out_cnt)
  pipeline32/1(q) -> sys_rst_cnt/1(out_cnt)
  Counter5/1 -> pipeline41/1(d)
  pipeline41/1(q) -> time_rst_cnt/1(out_cnt)
  [time_rst] -> Counter5/1
  [d80_adc0] -> bus_expand13/1(bus_in)
  cd_compensation0/2(dout) -> [hmc_data_p0]
  cd_compensation0/4(hmc_error) -> [hmc_error]
  [dvalid_tl_cd0] -> Gateway Out42/1, cd_compensation0/3(en)
  [sync_tl_cd0] -> Gateway Out41/1, cd_compensation0/1(sync_in)
  [dout_tl_cd0] -> Gateway Out44/1, cd_compensation0/2(din)
  [en_tl_cd0] -> cd_compensation0/5(load_val)
  [delay_tl_cd0] -> cd_compensation0/4(delay_val)
  Constant33/1 -> time_gen_cd/6(rd_misc_in)
  time_gen_cd/4(rd_misc_out) -> Terminator15/1
  [sync_tl_cd0] -> time_gen_cd/1(wr_sync_in)
  [dvalid_tl_cd0] -> time_gen_cd/2(wr_en)
  [hmc_sync_p0] -> time_gen_cd/4(rd_sync_in)
  [hmc_dvalid_p0] -> time_gen_cd/5(rd_en)
  time_gen_cd/1(rd_sync_out) -> [tg_rd_sync]
  time_gen_cd/2(rd_dvalid) -> [tg_rd_dvalid]
  [dvalid_tl_bs0] -> Gateway Out56/1, wb_prog_delay/4(en)
  [delay_tl_bs0] -> Gateway Out73/1, wb_prog_delay/2(delay_val)
  [delay_tl_sync0] -> Gateway Out55/1, wb_prog_delay/1(sync)
  [en_tl_bs0] -> Gateway Out72/1, wb_prog_delay/5(load_val)
  wb_prog_delay/2(data_out) -> [delay_d0]
  wb_prog_delay/3(dvalid) -> [delay_dv]
  [time80_tl_cd0] -> Slice9/1
  Slice9/1 -> time_gen_cd/3(wr_val_in)
  Constant35/1 -> Concat7/2
  time_gen_cd/3(rd_val_out) -> Concat7/1
  Concat7/1 -> [tg_rd_time_out]
  cd_compensation0/3(dvalid) -> [hmc_dvalid_p0]
  cd_compensation0/1(sync_out) -> [hmc_sync_p0]
  cd_compensation0/5(parity_error) -> [hmc_parity_pol0]
  wb_prog_delay/1(sync_out) -> [delay_sync]
  pipeline4/1(q) -> tl_cd_bs0/1(rst)
  pipeline1/1(q) -> tl_cd_bs0/2(current_time)
  pipeline42/1(q) -> Gateway Out74/1, tl_cd_bs0/3(load_value)
  pipeline45/1(q) -> Gateway Out52/1, tl_cd_bs0/4(sync_in)
  pipeline46/1(q) -> Gateway Out54/1, tl_cd_bs0/5(din)
  pipeline48/1(q) -> Gateway Out53/1, tl_cd_bs0/6(en)
  [clr_status] -> pipeline4/1(d)
  [tg_rd_time_out] -> pipeline1/1(d)
  [ld_val0] -> pipeline42/1(d)
  [tg_rd_sync] -> pipeline45/1(d)
  [tg_rd_dvalid] -> pipeline48/1(d)
  Constant34/1 -> tl_cd_bs0/7(misci)
  tl_cd_bs0/7(misco) -> Terminator12/1
  tl_cd_bs0/4(dout) -> [data_tl_bs0]
  tl_cd_bs0/6(time) -> Terminator13/1
  tl_cd_bs0/5(dvalid) -> [dvalid_tl_bs0]
  tl_cd_bs0/1(value) -> [delay_tl_bs0]
  tl_cd_bs0/3(sync_out) -> [delay_tl_sync0]
  tl_cd_bs0/2(enable) -> [en_tl_bs0]
  pipeline133/1(q) -> tl_cd_bs0/8(arm)
  pipeline134/1(q) -> tl_cd_bs0/9(load_immediate)
  pipeline135/1(q) -> tl_cd_bs0/10(load_time)
  [tl_cd0_arm] -> pipeline133/1(d)
  [tl_cd0_load_immediate] -> pipeline134/1(d)
  [tl_cd0_load_time] -> pipeline135/1(d)
  Gateway Out38/1 -> To Workspace49/1
  Gateway Out39/1 -> To Workspace28/1
  Gateway Out24/1 -> To Workspace31/1
  Gateway Out25/1 -> To Workspace32/1
  Gateway Out34/1 -> To Workspace45/1
  Gateway Out35/1 -> To Workspace46/1
  Gateway Out37/1 -> To Workspace47/1
  Gateway Out36/1 -> To Workspace48/1
  bus_expand7/8(lsb_out1) -> Gateway Out38/1
  bus_expand7/7(out2) -> Gateway Out39/1
  bus_expand7/6(out3) -> Gateway Out24/1
  bus_expand7/5(out4) -> Gateway Out25/1
  bus_expand7/4(out5) -> Gateway Out34/1
  bus_expand7/3(out6) -> Gateway Out35/1
  bus_expand7/2(out7) -> Gateway Out36/1
  bus_expand7/1(msb_out8) -> Gateway Out37/1
  [hmc_data_p0] -> bus_expand7/1(bus_in)
  Gateway Out59/1 -> To Workspace59/1
  [hmc_dvalid_p0] -> Gateway Out59/1
  Gateway Out60/1 -> To Workspace60/1
  [hmc_sync_p0] -> Gateway Out60/1
  bus_expand5/8(lsb_out1) -> Gateway Out19/1
  bus_expand5/7(out2) -> Gateway Out20/1
  bus_expand5/6(out3) -> Gateway Out21/1
  bus_expand5/5(out4) -> Gateway Out9/1
  bus_expand5/4(out5) -> Gateway Out17/1
  bus_expand5/3(out6) -> Gateway Out22/1
  bus_expand5/2(out7) -> Gateway Out23/1
  bus_expand5/1(msb_out8) -> Gateway Out18/1
  [delay_d0] -> bus_expand5/1(bus_in)
  Gateway Out18/1 -> To Workspace30/1
  Gateway Out23/1 -> To Workspace17/1
  Gateway Out22/1 -> To Workspace18/1
  Gateway Out17/1 -> To Workspace19/1
  Gateway Out9/1 -> To Workspace9/1
  Gateway Out21/1 -> To Workspace24/1
  Gateway Out20/1 -> To Workspace29/1
  Gateway Out19/1 -> To Workspace25/1
  Gateway Out58/1 -> To Workspace58/1
  [delay_dv] -> Gateway Out58/1
  Gateway Out61/1 -> To Workspace61/1
  [delay_sync] -> Gateway Out61/1
  Gateway Out41/1 -> To Workspace51/1
  Gateway Out42/1 -> To Workspace52/1
  Gateway Out44/1 -> To Workspace53/1
  Gateway Out52/1 -> To Workspace54/1
  Gateway Out53/1 -> To Workspace55/1
  Gateway Out54/1 -> To Workspace56/1
  Gateway Out55/1 -> To Workspace57/1
  Gateway Out56/1 -> To Workspace64/1
  Gateway Out57/1 -> To Workspace73/1
  [data_tl_bs0] -> Gateway Out57/1, wb_prog_delay/3(din)
  Gateway Out72/1 -> To Workspace74/1
  Gateway Out73/1 -> To Workspace75/1
  Gateway Out74/1 -> To Workspace76/1
  bus_expand3/1(msb_out8) -> pipeline49/1(d)  "hmc_out9"
  bus_expand3/8(lsb_out1) -> pipeline68/1(d)  "hmc_out16"
  pipeline68/1(q) -> cd_out/8(in_d07)
  pipeline67/1(q) -> cd_out/7(in_d06)
  pipeline61/1(q) -> cd_out/6(in_d05)
  pipeline60/1(q) -> cd_out/5(in_d04)
  pipeline54/1(q) -> cd_out/4(in_d03)
  pipeline53/1(q) -> cd_out/3(in_d02)
  pipeline50/1(q) -> cd_out/2(in_d01)
  pipeline49/1(q) -> cd_out/1(in_d00)
  bus_expand3/7(out2) -> pipeline67/1(d)
  bus_expand3/5(out4) -> pipeline60/1(d)
  bus_expand3/4(out5) -> pipeline54/1(d)
  bus_expand3/6(out3) -> pipeline61/1(d)
  bus_expand3/3(out6) -> pipeline53/1(d)
  bus_expand3/2(out7) -> pipeline50/1(d)
  pipeline70/1(q) -> cd_out/9(in_dvalid)
  pipeline69/1(q) -> cd_out/10(in_sync)
  pipeline72/1(q) -> cd_out/12(trig)
  pipeline71/1(q) -> cd_out/11(we)
  Logical4/1 -> pipeline71/1(d)
  [delay_sync] -> pipeline69/1(d), Logical4/2, pipeline72/1(d)
  [delay_d0] -> bus_expand3/1(bus_in)
  [delay_dv] -> Logical4/1, pipeline70/1(d)
  Gateway Out82/1 -> To Workspace85/1
  Gateway Out83/1 -> To Workspace78/1
  Gateway Out76/1 -> To Workspace79/1
  Gateway Out77/1 -> To Workspace80/1
  Gateway Out78/1 -> To Workspace81/1
  Gateway Out79/1 -> To Workspace82/1
  Gateway Out81/1 -> To Workspace83/1
  Gateway Out80/1 -> To Workspace84/1
  bus_expand9/8(lsb_out1) -> Gateway Out82/1
  bus_expand9/7(out2) -> Gateway Out83/1
  bus_expand9/6(out3) -> Gateway Out76/1
  bus_expand9/5(out4) -> Gateway Out77/1
  bus_expand9/4(out5) -> Gateway Out78/1
  bus_expand9/3(out6) -> Gateway Out79/1
  bus_expand9/2(out7) -> Gateway Out80/1
  bus_expand9/1(msb_out8) -> Gateway Out81/1
  [data_tl_bs0] -> bus_expand9/1(bus_in)
  [hmc_data_p0] -> Delay20/1
  Delay20/1 -> [tg_data_p0]
  [tg_data_p0] -> pipeline46/1(d)
  [hmc_parity_pol1] -> Terminator1/1
  bus_expand8/1(msb_out8) -> pipeline167/1(d)  "hmc_out9"
  bus_expand8/8(lsb_out1) -> pipeline136/1(d)  "hmc_out16"
  bus_expand8/7(out2) -> pipeline132/1(d)
  bus_expand8/5(out4) -> pipeline93/1(d)
  bus_expand8/4(out5) -> pipeline92/1(d)
  bus_expand8/6(out3) -> pipeline131/1(d)
  bus_expand8/3(out6) -> pipeline91/1(d)
  bus_expand8/2(out7) -> pipeline90/1(d)
  pipeline140/1(q) -> hmc_out/12(trig)
  pipeline139/1(q) -> hmc_out/11(we)
  Logical13/1 -> pipeline139/1(d)
  [hmc_sync_p0] -> pipeline140/1(d), Logical13/2, pipeline137/1(d)
  [hmc_dvalid_p0] -> pipeline138/1(d), Logical13/1
  pipeline167/1(q) -> hmc_out/1(in_d0)
  pipeline90/1(q) -> hmc_out/2(in_d1)
  pipeline91/1(q) -> hmc_out/3(in_d2)
  pipeline92/1(q) -> hmc_out/4(in_d3)
  pipeline93/1(q) -> hmc_out/5(in_d4)
  pipeline131/1(q) -> hmc_out/6(in_d5)
  pipeline132/1(q) -> hmc_out/7(in_d6)
  pipeline136/1(q) -> hmc_out/8(in_d7)
  pipeline138/1(q) -> hmc_out/9(in_dv)
  pipeline137/1(q) -> hmc_out/10(in_sync)
  pipeline142/1(q) -> tl_cd1/1(rst)
  [ld_val1] -> pipeline143/1(d)
  [d80_adc0] -> pipeline144/1(d)
  pipeline141/1(q) -> tl_cd1/2(current_time)
  pipeline143/1(q) -> tl_cd1/3(load_value)
  pipeline147/1(q) -> tl_cd1/4(sync_in)
  pipeline144/1(q) -> tl_cd1/5(din)
  pipeline145/1(q) -> tl_cd1/6(en)
  pipeline148/1(q) -> tl_cd1/9(load_immediate)
  pipeline146/1(q) -> tl_cd1/8(arm)
  pipeline149/1(q) -> tl_cd1/10(load_time)
  [tl_cd1_arm] -> pipeline146/1(d)
  [tl_cd1_load_immediate] -> pipeline148/1(d)
  [tl_cd1_load_time] -> pipeline149/1(d)
  Constant17/1 -> tl_cd1/7(misci)
  tl_cd1/1(value) -> [delay_tl_cd1]
  tl_cd1/2(enable) -> [en_tl_cd1]
  tl_cd1/3(sync_out) -> [sync_tl_cd1]
  tl_cd1/4(dout) -> [dout_tl_cd1]
  tl_cd1/5(dvalid) -> [dvalid_tl_cd1]
  tl_cd1/6(time) -> [time80_tl_cd1]
  tl_cd1/7(misco) -> Terminator3/1
  cd_compensation1/5(parity_error) -> [hmc_parity_pol1]
  cd_compensation1/4(hmc_error) -> Terminator20/1
  [delay_tl_cd1] -> cd_compensation1/4(delay_val)
  [en_tl_cd1] -> cd_compensation1/5(load_val)
  [sync_tl_cd1] -> cd_compensation1/1(sync_in)
  [dout_tl_cd1] -> cd_compensation1/2(din)
  [dvalid_tl_cd1] -> cd_compensation1/3(en)
  cd_compensation1/1(sync_out) -> [hmc_sync_p1]
  cd_compensation1/2(dout) -> [hmc_data_p1]
  cd_compensation1/3(dvalid) -> [hmc_dvalid_p1]
  [hmc_data_p1] -> Delay2/1
  Delay2/1 -> [tg_data_p1]
  pipeline151/1(q) -> tl_cd_bs1/1(rst)
  pipeline150/1(q) -> tl_cd_bs1/2(current_time)
  pipeline152/1(q) -> tl_cd_bs1/3(load_value)
  pipeline153/1(q) -> tl_cd_bs1/4(sync_in)
  pipeline154/1(q) -> tl_cd_bs1/5(din)
  pipeline155/1(q) -> tl_cd_bs1/6(en)
  [clr_status] -> pipeline151/1(d)
  [tg_rd_time_out] -> pipeline150/1(d)
  [ld_val1] -> pipeline152/1(d)
  [tg_rd_sync] -> pipeline153/1(d)
  [tg_rd_dvalid] -> pipeline155/1(d)
  [tg_data_p1] -> pipeline154/1(d)
  Constant36/1 -> tl_cd_bs1/7(misci)
  pipeline156/1(q) -> tl_cd_bs1/8(arm)
  pipeline157/1(q) -> tl_cd_bs1/9(load_immediate)
  pipeline158/1(q) -> tl_cd_bs1/10(load_time)
  [tl_cd1_load_time] -> pipeline158/1(d)
  [tl_cd1_load_immediate] -> pipeline157/1(d)
  [tl_cd1_arm] -> pipeline156/1(d)
  tl_cd_bs1/7(misco) -> Terminator7/1
  tl_cd_bs1/4(dout) -> [data_tl_bs1]
  tl_cd_bs1/6(time) -> Terminator5/1
  tl_cd_bs1/5(dvalid) -> [dvalid_tl_bs1]
  tl_cd_bs1/1(value) -> [delay_tl_bs1]
  tl_cd_bs1/3(sync_out) -> [delay_tl_sync1]
  tl_cd_bs1/2(enable) -> [en_tl_bs1]
  [delay_tl_sync1] -> wb_prog_delay1/1(sync)
  [delay_tl_bs1] -> wb_prog_delay1/2(delay_val)
  [en_tl_bs1] -> wb_prog_delay1/5(load_val)
  [data_tl_bs1] -> wb_prog_delay1/3(din)
  [dvalid_tl_bs1] -> wb_prog_delay1/4(en)
  wb_prog_delay1/2(data_out) -> [delay_d1]
  wb_prog_delay1/1(sync_out) -> [delay_sync_p1]
  bus_expand10/1(msb_out8) -> pipeline159/1(d)  "hmc_out9"
  bus_expand10/8(lsb_out1) -> pipeline166/1(d)  "hmc_out16"
  pipeline166/1(q) -> cd_out1/8(in_d07)
  pipeline165/1(q) -> cd_out1/7(in_d06)
  pipeline164/1(q) -> cd_out1/6(in_d05)
  pipeline163/1(q) -> cd_out1/5(in_d04)
  pipeline162/1(q) -> cd_out1/4(in_d03)
  pipeline161/1(q) -> cd_out1/3(in_d02)
  pipeline160/1(q) -> cd_out1/2(in_d01)
  pipeline159/1(q) -> cd_out1/1(in_d00)
  bus_expand10/7(out2) -> pipeline165/1(d)
  bus_expand10/5(out4) -> pipeline163/1(d)
  bus_expand10/4(out5) -> pipeline162/1(d)
  bus_expand10/6(out3) -> pipeline164/1(d)
  bus_expand10/3(out6) -> pipeline161/1(d)
  bus_expand10/2(out7) -> pipeline160/1(d)
  pipeline169/1(q) -> cd_out1/9(in_dvalid)
  pipeline168/1(q) -> cd_out1/10(in_sync)
  pipeline171/1(q) -> cd_out1/12(trig)
  pipeline170/1(q) -> cd_out1/11(we)
  Logical16/1 -> pipeline170/1(d)
  [delay_sync_p1] -> pipeline171/1(d), Logical16/2, pipeline168/1(d)
  [delay_d1] -> bus_expand10/1(bus_in)
  [delay_dv_p1] -> pipeline169/1(d), Logical16/1
  [d80_adc1] -> Terminator17/1
  wb_prog_delay1/3(dvalid) -> [delay_dv_p1]
  [hmc_data_p0] -> bus_expand8/1(bus_in)
  [tvg_adc_en] -> impulse_gen1/1(tvg_en), impulse_gen0/1(tvg_en)
